simulink model "Example_13_1_3_2"  (R2018a)
settings: Solver=FixedStepAuto  StartTime=0.0  StopTime=0.5  FixedStep=0.001  RelTol=1e-3
settings Model: Creator=ahmed  LastModifiedBy=ahmed

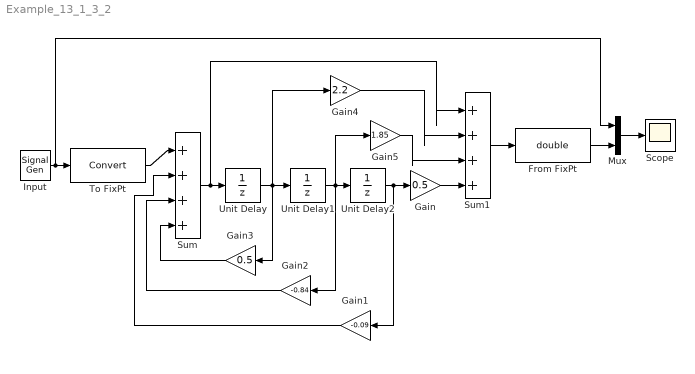
== system Example_13_1_3_2 ==
  From FixPt : DataTypeConversion  OutDataTypeStr=double
  Gain : Gain  Gain=0.5
  Gain1 : Gain  Gain=-0.09
  Gain2 : Gain  Gain=-0.84
  Gain3 : Gain  Gain=0.5
  Gain4 : Gain  Gain=2.2
  Gain5 : Gain  Gain=1.85
  Input : SignalGenerator  WaveForm=square  Frequency=2
  Mux : Mux  Inputs=2
  Scope : Scope
  Sum : Sum  Inputs=|++++
  Sum1 : Sum  Inputs=|++++
  To FixPt : DataTypeConversion
  Unit Delay : UnitDelay  SampleTime=-1
  Unit Delay1 : UnitDelay  SampleTime=-1
  Unit Delay2 : UnitDelay  SampleTime=-1
  wires:
  To FixPt/1 -> Sum/1
  Sum/1 -> Sum1/1, Unit Delay/1
  Unit Delay/1 -> Gain4/1, Unit Delay1/1, Gain3/1
  Unit Delay1/1 -> Gain5/1, Gain2/1, Unit Delay2/1
  Unit Delay2/1 -> Gain1/1, Gain/1
  Gain/1 -> Sum1/4
  Gain3/1 -> Sum/4
  Gain2/1 -> Sum/3
  Gain1/1 -> Sum/2
  Gain5/1 -> Sum1/3
  Gain4/1 -> Sum1/2
  Sum1/1 -> From FixPt/1
  From FixPt/1 -> Mux/2
  Input/1 -> Mux/1, To FixPt/1
  Mux/1 -> Scope/1
